simulink model "RM3ControlSim"  (R2015b)
settings: Solver=ode4  StartTime=0  StopTime=400  FixedStep=0.1  MaxStep=0.1  RelTol=1e-3
values from neighbouring files (symbols this model uses):
  simu = simulationClass()    [wecSimInputFile.m]
  waves = waveClass('irregular')    [wecSimInputFile.m]
undefined symbols (not defined in the file or in its folder): body, constraint, plant, pto, X, Y, Z
libraries: nesl_utility x72, vrlib x24, sm_lib x24, WECSim_Lib x3, simulink x2
(part 4 of 6)

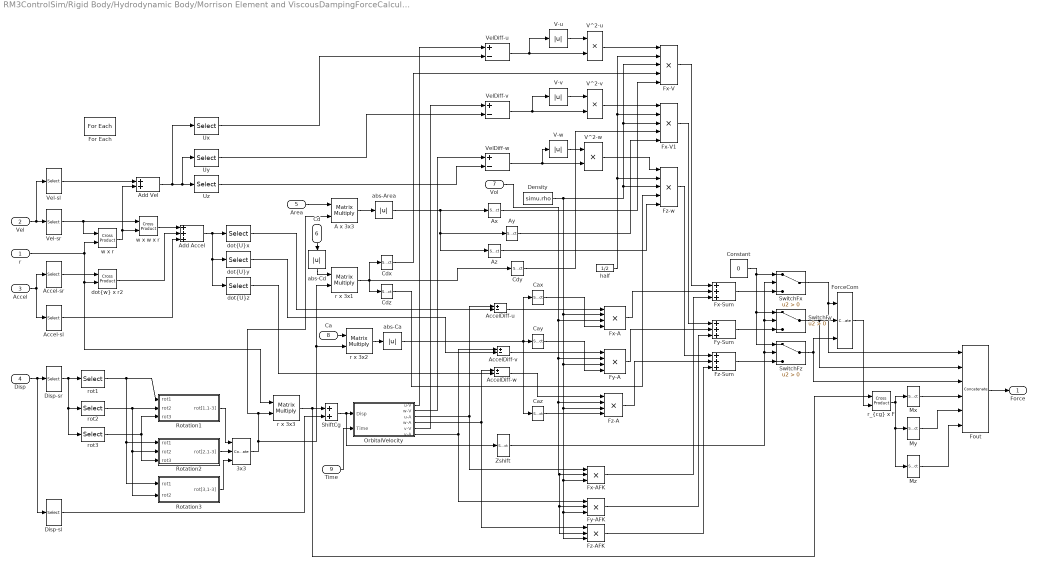
== system RM3ControlSim/Rigid Body/Hydrodynamic Body/Morrison Element and ViscousDampingForceCalculation/Morrison Element Variant Subsystem/Morrison Element On/Regular Wave Morison Force/MorrisonElements ==
  r : Inport  Partition=on  PartitionDimension=1  PartitionWidth=1
  Vel : Inport  Port=2
  Accel : Inport  Port=3
  Disp : Inport  Port=4
  Area : Inport  Port=5  Partition=on  PartitionDimension=1  PartitionWidth=1
  Cd : Inport  Port=6  Partition=on  PartitionDimension=1  PartitionWidth=1
  Vol : Inport  Port=7  Partition=on  PartitionDimension=1  PartitionWidth=1
  Ca : Inport  Port=8  Partition=on  PartitionDimension=1  PartitionWidth=1
  Time : Inport  Port=9
  3x3 : Concatenate  NumInputs=3  Mode=Multidimensional array
  A x 3x3 : Product  Multiplication=Matrix(*)
  Accel-sl : Selector  InputPortWidth=6  IndexOptions=Index vector (dialog)  Indices=[1 2 3]  OutputSizes=1
  Accel-sr : Selector  InputPortWidth=6  IndexOptions=Index vector (dialog)  Indices=[4 5 6]  OutputSizes=1
  AccelDiff-u : Sum  Inputs=+-
  AccelDiff-v : Sum  Inputs=+-
  AccelDiff-w : Sum  Inputs=+-
  Add Accel : Sum  Inputs=+++
  Add Vel : Sum
  Ax : Selector  InputPortWidth=3  IndexOptions=Index vector (dialog)  Indices=[1]  OutputSizes=1
  Ay : Selector  InputPortWidth=3  IndexOptions=Index vector (dialog)  Indices=[2]  OutputSizes=1
  Az : Selector  InputPortWidth=3  IndexOptions=Index vector (dialog)  Indices=[3]  OutputSizes=1
  Cax : Selector  InputPortWidth=3  IndexOptions=Index vector (dialog)  Indices=[1]  OutputSizes=1
  Cay : Selector  InputPortWidth=3  IndexOptions=Index vector (dialog)  Indices=[2]  OutputSizes=1
  Caz : Selector  InputPortWidth=3  IndexOptions=Index vector (dialog)  Indices=[3]  OutputSizes=1
  Cdx : Selector  InputPortWidth=3  IndexOptions=Index vector (dialog)  Indices=[1]  OutputSizes=1
  Cdy : Selector  InputPortWidth=3  IndexOptions=Index vector (dialog)  Indices=[2]  OutputSizes=1
  Cdz : Selector  InputPortWidth=3  IndexOptions=Index vector (dialog)  Indices=[3]  OutputSizes=1
  Constant : Constant  Value=0
  Density : Constant  Value=simu.rho
  Disp-sl : Selector  InputPortWidth=6  IndexOptions=Index vector (dialog)  Indices=[1 2 3]  OutputSizes=1
  Disp-sr : Selector  InputPortWidth=6  IndexOptions=Index vector (dialog)  Indices=[4 5 6]  OutputSizes=1
  For Each : ForEach  DisableCoverage=on  IndexMode=One-based
  ForceCom : Concatenate  NumInputs=3  ConcatenateDimension=2
  Fout : Concatenate  NumInputs=6  Mode=Multidimensional array  ConcatenateDimension=2
  Fx-A : Product  Inputs=4
  Fx-AFK : Product  Inputs=3
  Fx-Sum : Sum  Inputs=+++
  Fx-V : Product  Inputs=5
  Fx-V1 : Product  Inputs=5
  Fy-A : Product  Inputs=4
  Fy-AFK : Product  Inputs=3
  Fy-Sum : Sum  Inputs=+++
  Fz-A : Product  Inputs=4
  Fz-AFK : Product  Inputs=3
  Fz-Sum : Sum  Inputs=+++
  Fz-w : Product  Inputs=5
  Mx : Selector  InputPortWidth=3  IndexOptions=Index vector (dialog)  Indices=[1]  OutputSizes=1
  My : Selector  InputPortWidth=3  IndexOptions=Index vector (dialog)  Indices=[2]  OutputSizes=1
  Mz : Selector  InputPortWidth=3  IndexOptions=Index vector (dialog)  Indices=[3]  OutputSizes=1
  OrbitalVelocity : Subsystem
  Rotation1 : Subsystem
  Rotation2 : Subsystem
  Rotation3 : Subsystem
  ShiftCg : Sum
  SwitchFx : Switch  Criteria=u2 > Threshold
  SwitchFy : Switch  Criteria=u2 > Threshold
  SwitchFz : Switch  Criteria=u2 > Threshold
  Ux : Selector  InputPortWidth=3  IndexOptions=Index vector (dialog)  Indices=[1]  OutputSizes=1
  Uy : Selector  InputPortWidth=3  IndexOptions=Index vector (dialog)  Indices=[2]  OutputSizes=1
  Uz : Selector  InputPortWidth=3  IndexOptions=Index vector (dialog)  Indices=[3]  OutputSizes=1
  V-u : Abs
  V-v : Abs
  V-w : Abs
  V^2-u : Product
  V^2-v : Product
  V^2-w : Product
  Vel-sl : Selector  InputPortWidth=6  IndexOptions=Index vector (dialog)  Indices=[1 2 3]  OutputSizes=1
  "Vel-sr " : Selector  InputPortWidth=6  IndexOptions=Index vector (dialog)  Indices=[4 5 6]  OutputSizes=1
  VelDiff-u : Sum  Inputs=+-
  VelDiff-v : Sum  Inputs=+-
  VelDiff-w : Sum  Inputs=+-
  Zshift : Selector  InputPortWidth=3  IndexOptions=Index vector (dialog)  Indices=[3]  OutputSizes=1
  abs-Area : Abs
  abs-Ca : Abs
  abs-Cd : Abs
  "dot{U}x" : Selector  InputPortWidth=3  IndexOptions=Index vector (dialog)  Indices=[1]  OutputSizes=1
  "dot{U}y" : Selector  InputPortWidth=3  IndexOptions=Index vector (dialog)  Indices=[2]  OutputSizes=1
  "dot{U}z" : Selector  InputPortWidth=3  IndexOptions=Index vector (dialog)  Indices=[3]  OutputSizes=1
  "dot{w} x r2" : vrlib/Utilities/Cross Product
  half : Constant  Value=1/2
  r x 3x1 : Product  Multiplication=Matrix(*)
  r x 3x2 : Product  Multiplication=Matrix(*)
  r x 3x3 : Product  Multiplication=Matrix(*)
  "r_{cg} x F" : vrlib/Utilities/Cross Product
  rot1 : Selector  InputPortWidth=3  IndexOptions=Index vector (dialog)  Indices=[1]  OutputSizes=1
  rot2 : Selector  InputPortWidth=3  IndexOptions=Index vector (dialog)  Indices=[2]  OutputSizes=1
  rot3 : Selector  InputPortWidth=3  IndexOptions=Index vector (dialog)  Indices=[3]  OutputSizes=1
  w x r : vrlib/Utilities/Cross Product
  w x w x r : vrlib/Utilities/Cross Product
  Force : Outport  PortDimensions=[1 6]  ConcatenationDimension=1
  wires:
  Time/1 -> OrbitalVelocity/2(Time)
  abs-Cd/1 -> r x 3x1/1
  abs-Ca/1 -> Caz/1, Cay/1, Cax/1
  V-w/1 -> V^2-w/1
  Constant/1 -> SwitchFx/1, SwitchFz/1, SwitchFy/1
  Fx-V1/1 -> Fy-Sum/1
  Fy-A/1 -> Fy-Sum/2
  Cay/1 -> Fy-A/4
  AccelDiff-v/1 -> Fy-A/1
  Fy-AFK/1 -> Fy-Sum/3
  Fy-Sum/1 -> SwitchFy/3
  SwitchFy/1 -> ForceCom/2, Fout/2
  Cdy/1 -> Fx-V1/4
  Ay/1 -> Fx-V1/5
  OrbitalVelocity/5(v-V) -> VelDiff-v/1
  VelDiff-v/1 -> V^2-v/2, V-v/1
  V-v/1 -> V^2-v/1
  V^2-v/1 -> Fx-V1/1
  OrbitalVelocity/6(v-A) -> Fy-AFK/1, AccelDiff-v/1
  r x 3x2/1 -> abs-Ca/1
  Ca/1 -> r x 3x2/1
  r x 3x1/1 -> Cdx/1, Cdz/1, Cdy/1
  Cd/1 -> abs-Cd/1
  Cax/1 -> Fx-A/4
  Caz/1 -> Fz-A/4
  Fout/1 -> Force/1
  ForceCom/1 -> "r_{cg} x F"/2
  abs-Area/1 -> Ax/1, Az/1, Ay/1
  A x 3x3/1 -> abs-Area/1
  Cdz/1 -> Fz-w/4
  Cdx/1 -> Fx-V/4
  Ax/1 -> Fx-V/5
  Area/1 -> A x 3x3/1
  Az/1 -> Fz-w/5
  Fz-Sum/1 -> SwitchFz/3
  Fx-Sum/1 -> SwitchFx/3
  SwitchFx/1 -> ForceCom/1, Fout/1
  SwitchFz/1 -> Fout/3, ForceCom/3
  Zshift/1 -> SwitchFz/2, SwitchFx/2, SwitchFy/2
  VelDiff-u/1 -> V^2-u/2, V-u/1
  V-u/1 -> V^2-u/1
  3x3/1 -> r x 3x1/2, r x 3x2/2, r x 3x3/2, A x 3x3/2
  Mz/1 -> Fout/6
  My/1 -> Fout/5
  Mx/1 -> Fout/4
  "r_{cg} x F"/1 -> Mx/1, My/1, Mz/1
  Fz-AFK/1 -> Fz-Sum/3
  Fz-A/1 -> Fz-Sum/2
  Fz-w/1 -> Fz-Sum/1
  Fx-AFK/1 -> Fx-Sum/3
  Fx-A/1 -> Fx-Sum/2
  Fx-V/1 -> Fx-Sum/1
  OrbitalVelocity/4(w-A) -> AccelDiff-w/1, Fz-AFK/1
  AccelDiff-w/1 -> Fz-A/1
  Vol/1 -> Fx-A/3, Fz-A/2, Fx-AFK/2, Fz-AFK/2, Fy-AFK/2, Fy-A/2
  AccelDiff-u/1 -> Fx-A/1
  V^2-w/1 -> Fz-w/1
  Density/1 -> Fx-V/3, Fx-V1/3, Fz-w/3, Fx-A/2, Fz-A/3, Fx-AFK/3, Fz-AFK/3, Fy-AFK/3, Fy-A/3
  half/1 -> Fx-V/2, Fx-V1/2, Fz-w/2
  V^2-u/1 -> Fx-V/1
  VelDiff-w/1 -> V^2-w/2, V-w/1
  OrbitalVelocity/2(w-V) -> VelDiff-w/1
  OrbitalVelocity/1(u-V) -> VelDiff-u/1
  Uz/1 -> VelDiff-w/2
  Ux/1 -> VelDiff-u/2
  Uy/1 -> VelDiff-v/2
  Add Vel/1 -> Ux/1, Uz/1, Uy/1
  "dot{U}z"/1 -> AccelDiff-w/2
  OrbitalVelocity/3(u-A) -> Fx-AFK/1, AccelDiff-u/1
  "dot{U}x"/1 -> AccelDiff-u/2
  "dot{U}y"/1 -> AccelDiff-v/2
  ShiftCg/1 -> OrbitalVelocity/1(Disp), Zshift/1
  Disp-sl/1 -> ShiftCg/2
  r x 3x3/1 -> ShiftCg/1, "r_{cg} x F"/1
  Rotation3/1(rot[3,1-3]) -> 3x3/3
  Rotation1/1(rot[1,1-3]) -> 3x3/1
  Rotation2/1(rot[2,1-3]) -> 3x3/2
  rot2/1 -> Rotation1/2(rot2), Rotation2/2(rot2), Rotation3/2(rot2)
  rot1/1 -> Rotation1/1(rot1), Rotation2/1(rot1), Rotation3/1(rot1)
  rot3/1 -> Rotation1/3(rot3), Rotation2/3(rot3)
  Disp-sr/1 -> rot1/1, rot2/1, rot3/1
  Disp/1 -> Disp-sr/1, Disp-sl/1
  Vel-sl/1 -> Add Vel/1
  Add Accel/1 -> "dot{U}x"/1, "dot{U}y"/1, "dot{U}z"/1
  Accel-sl/1 -> Add Accel/3
  "dot{w} x r2"/1 -> Add Accel/2
  Accel-sr/1 -> "dot{w} x r2"/1
  Accel/1 -> Accel-sr/1, Accel-sl/1
  r/1 -> w x r/2, "dot{w} x r2"/2, r x 3x3/1
  "Vel-sr "/1 -> w x r/1, w x w x r/1
  w x w x r/1 -> Add Accel/1
  w x r/1 -> w x w x r/2, Add Vel/2
  Vel/1 -> "Vel-sr "/1, Vel-sl/1

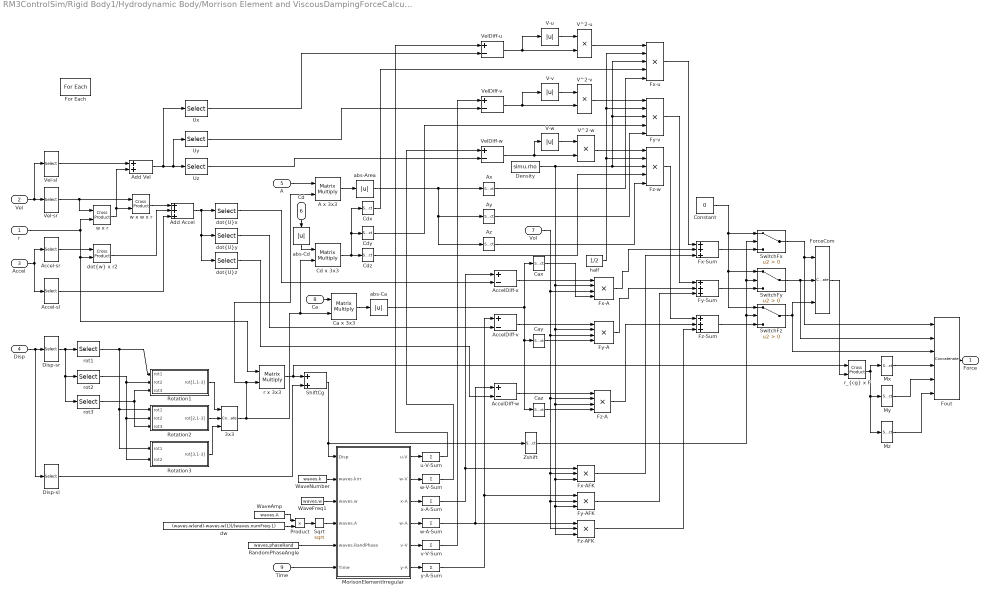
== system RM3ControlSim/Rigid Body1/Hydrodynamic Body/Morrison Element and ViscousDampingForceCalculation/Morrison Element Variant Subsystem/Morrison Element On/Irregular Wave Morison Force/MorrisonElements ==
  r : Inport  Partition=on  PartitionDimension=1  PartitionWidth=1
  Vel : Inport  Port=2
  Accel : Inport  Port=3
  Disp : Inport  Port=4
  A : Inport  Port=5  Partition=on  PartitionDimension=1  PartitionWidth=1
  Cd : Inport  Port=6  Partition=on  PartitionDimension=1  PartitionWidth=1
  Vol : Inport  Port=7  Partition=on  PartitionDimension=1  PartitionWidth=1
  Ca : Inport  Port=8  Partition=on  PartitionDimension=1  PartitionWidth=1
  Time : Inport  Port=9
  3x3 : Concatenate  NumInputs=3  Mode=Multidimensional array
  A x 3x3 : Product  Multiplication=Matrix(*)
  Accel-sl : Selector  InputPortWidth=6  IndexOptions=Index vector (dialog)  Indices=[1 2 3]  OutputSizes=1
  Accel-sr : Selector  InputPortWidth=6  IndexOptions=Index vector (dialog)  Indices=[4 5 6]  OutputSizes=1
  AccelDiff-v : Sum  Inputs=+-
  AccelDiff-w : Sum  Inputs=+-
  AccelDiff-x : Sum  Inputs=+-
  Add Accel : Sum  Inputs=+++
  Add Vel : Sum
  Ax : Selector  InputPortWidth=3  IndexOptions=Index vector (dialog)  Indices=[1]  OutputSizes=1
  Ay : Selector  InputPortWidth=3  IndexOptions=Index vector (dialog)  Indices=[2]  OutputSizes=1
  Az : Selector  InputPortWidth=3  IndexOptions=Index vector (dialog)  Indices=[3]  OutputSizes=1
  Ca x 3x3 : Product  Multiplication=Matrix(*)
  Cax : Selector  InputPortWidth=3  IndexOptions=Index vector (dialog)  Indices=[1]  OutputSizes=1
  Cay : Selector  InputPortWidth=3  IndexOptions=Index vector (dialog)  Indices=[2]  OutputSizes=1
  Caz : Selector  InputPortWidth=3  IndexOptions=Index vector (dialog)  Indices=[3]  OutputSizes=1
  Cd x 3x3 : Product  Multiplication=Matrix(*)
  Cdx : Selector  InputPortWidth=3  IndexOptions=Index vector (dialog)  Indices=[1]  OutputSizes=1
  Cdy : Selector  InputPortWidth=3  IndexOptions=Index vector (dialog)  Indices=[2]  OutputSizes=1
  Cdz : Selector  InputPortWidth=3  IndexOptions=Index vector (dialog)  Indices=[3]  OutputSizes=1
  Constant : Constant  Value=0
  Density : Constant  Value=simu.rho
  Disp-sl : Selector  InputPortWidth=6  IndexOptions=Index vector (dialog)  Indices=[1 2 3]  OutputSizes=1
  Disp-sr : Selector  InputPortWidth=6  IndexOptions=Index vector (dialog)  Indices=[4 5 6]  OutputSizes=1
  For Each : ForEach  DisableCoverage=on  IndexMode=One-based
  ForceCom : Concatenate  NumInputs=3  ConcatenateDimension=2
  Fout : Concatenate  NumInputs=6  Mode=Multidimensional array  ConcatenateDimension=2
  Fx-A : Product  Inputs=4
  Fx-AFK : Product  Inputs=3
  Fx-Sum : Sum  Inputs=+++
  Fx-u : Product  Inputs=5
  Fy-A : Product  Inputs=4
  Fy-AFK : Product  Inputs=3
  Fy-Sum : Sum  Inputs=+++
  Fy-v : Product  Inputs=5
  Fz-A : Product  Inputs=4
  Fz-AFK : Product  Inputs=3
  Fz-Sum : Sum  Inputs=+++
  Fz-w : Product  Inputs=5
  MorisonElementIrregular : Subsystem  TreatAsAtomicUnit=on
  Mx : Selector  InputPortWidth=3  IndexOptions=Index vector (dialog)  Indices=[1]  OutputSizes=1
  My : Selector  InputPortWidth=3  IndexOptions=Index vector (dialog)  Indices=[2]  OutputSizes=1
  Mz : Selector  InputPortWidth=3  IndexOptions=Index vector (dialog)  Indices=[3]  OutputSizes=1
  Product : Product
  RandomPhaseAngle : Constant  Value=waves.phaseRand  VectorParams1D=off
  Rotation1 : Subsystem
  Rotation2 : Subsystem
  Rotation3 : Subsystem
  ShiftCg : Sum
  Sqrt : Sqrt  SaturateOnIntegerOverflow=on
  SwitchFx : Switch  Criteria=u2 > Threshold
  SwitchFy : Switch  Criteria=u2 > Threshold
  SwitchFz : Switch  Criteria=u2 > Threshold
  Ux : Selector  InputPortWidth=3  IndexOptions=Index vector (dialog)  Indices=[1]  OutputSizes=1
  Uy : Selector  InputPortWidth=3  IndexOptions=Index vector (dialog)  Indices=[2]  OutputSizes=1
  Uz : Selector  InputPortWidth=3  IndexOptions=Index vector (dialog)  Indices=[3]  OutputSizes=1
  V-u : Abs
  V-v : Abs
  V-w : Abs
  V^2-u : Product
  V^2-v : Product
  V^2-w : Product
  Vel-sl : Selector  InputPortWidth=6  IndexOptions=Index vector (dialog)  Indices=[1 2 3]  OutputSizes=1
  "Vel-sr " : Selector  InputPortWidth=6  IndexOptions=Index vector (dialog)  Indices=[4 5 6]  OutputSizes=1
  VelDiff-u : Sum  Inputs=+-
  VelDiff-v : Sum  Inputs=+-
  VelDiff-w : Sum  Inputs=+-
  WaveAmp : Constant  Value=waves.A  VectorParams1D=off
  WaveFreq1 : Constant  Value=waves.w  VectorParams1D=off
  WaveNumber : Constant  Value=waves.k  VectorParams1D=off
  Zshift : Selector  InputPortWidth=3  IndexOptions=Index vector (dialog)  Indices=[3]  OutputSizes=1
  abs-Area : Abs
  abs-Ca : Abs
  abs-Cd : Abs
  "dot{U}x" : Selector  InputPortWidth=3  IndexOptions=Index vector (dialog)  Indices=[1]  OutputSizes=1
  "dot{U}y" : Selector  InputPortWidth=3  IndexOptions=Index vector (dialog)  Indices=[2]  OutputSizes=1
  "dot{U}z" : Selector  InputPortWidth=3  IndexOptions=Index vector (dialog)  Indices=[3]  OutputSizes=1
  "dot{w} x r2" : vrlib/Utilities/Cross Product
  dw : Constant  Value=(waves.w(end)-waves.w(1))/(waves.numFreq-1)  VectorParams1D=off
  half : Constant  Value=1/2
  r x 3x3 : Product  Multiplication=Matrix(*)
  "r_{cg} x F" : vrlib/Utilities/Cross Product
  rot1 : Selector  InputPortWidth=3  IndexOptions=Index vector (dialog)  Indices=[1]  OutputSizes=1
  rot2 : Selector  InputPortWidth=3  IndexOptions=Index vector (dialog)  Indices=[2]  OutputSizes=1
  rot3 : Selector  InputPortWidth=3  IndexOptions=Index vector (dialog)  Indices=[3]  OutputSizes=1
  u-V-Sum : Sum  Inputs=+  CollapseMode=Specified dimension
  v-V-Sum : Sum  Inputs=+  CollapseMode=Specified dimension
  w x r : vrlib/Utilities/Cross Product
  w x w x r : vrlib/Utilities/Cross Product
  w-A-Sum : Sum  Inputs=+  CollapseMode=Specified dimension
  w-V-Sum : Sum  Inputs=+  CollapseMode=Specified dimension
  x-A-Sum : Sum  Inputs=+  CollapseMode=Specified dimension
  y-A-Sum : Sum  Inputs=+  CollapseMode=Specified dimension
  Force : Outport  PortDimensions=[1 6]  ConcatenationDimension=1
  wires:
  Time/1 -> MorisonElementIrregular/6(Time)
  abs-Cd/1 -> Cd x 3x3/1
  abs-Ca/1 -> Cay/1, Caz/1, Cax/1
  Fy-AFK/1 -> Fy-Sum/3
  Fy-A/1 -> Fy-Sum/2
  AccelDiff-v/1 -> Fy-A/1
  Cay/1 -> Fy-A/4
  y-A-Sum/1 -> AccelDiff-v/1, Fy-AFK/1
  Fy-v/1 -> Fy-Sum/1
  Fy-Sum/1 -> SwitchFy/3
  SwitchFy/1 -> ForceCom/2, Fout/2
  Cdy/1 -> Fy-v/4
  Ay/1 -> Fy-v/5
  V^2-v/1 -> Fy-v/1
  v-V-Sum/1 -> VelDiff-v/1
  V-v/1 -> V^2-v/1
  VelDiff-v/1 -> V^2-v/2, V-v/1
  V-w/1 -> V^2-w/1
  MorisonElementIrregular/6(y-A) -> y-A-Sum/1
  MorisonElementIrregular/5(v-V) -> v-V-Sum/1
  V-u/1 -> V^2-u/1
  MorisonElementIrregular/4(w-A) -> w-A-Sum/1
  MorisonElementIrregular/3(x-A) -> x-A-Sum/1
  MorisonElementIrregular/2(w-V) -> w-V-Sum/1
  Sqrt/1 -> MorisonElementIrregular/4(waves.A)
  Product/1 -> Sqrt/1
  dw/1 -> Product/2
  WaveAmp/1 -> Product/1
  MorisonElementIrregular/1(u-V) -> u-V-Sum/1
  RandomPhaseAngle/1 -> MorisonElementIrregular/5(waves.RandPhase)
  WaveFreq1/1 -> MorisonElementIrregular/3(waves.w)
  WaveNumber/1 -> MorisonElementIrregular/2(waves.kirr)
  Ca x 3x3/1 -> abs-Ca/1
  Ca/1 -> Ca x 3x3/1
  Cd x 3x3/1 -> Cdx/1, Cdy/1, Cdz/1
  Cd/1 -> abs-Cd/1
  Cax/1 -> Fx-A/4
  Caz/1 -> Fz-A/4
  Fout/1 -> Force/1
  ForceCom/1 -> "r_{cg} x F"/2
  abs-Area/1 -> Ax/1, Az/1, Ay/1
  A x 3x3/1 -> abs-Area/1
  Cdz/1 -> Fz-w/4
  Cdx/1 -> Fx-u/4
  Ax/1 -> Fx-u/5
  A/1 -> A x 3x3/1
  Az/1 -> Fz-w/5
  Fz-Sum/1 -> SwitchFz/3
  Fx-Sum/1 -> SwitchFx/3
  SwitchFx/1 -> ForceCom/1, Fout/1
  SwitchFz/1 -> Fout/3, ForceCom/3
  Zshift/1 -> SwitchFz/2, SwitchFx/2, SwitchFy/2
  VelDiff-u/1 -> V^2-u/2, V-u/1
  3x3/1 -> Cd x 3x3/2, Ca x 3x3/2, r x 3x3/2, A x 3x3/2
  Mz/1 -> Fout/6
  My/1 -> Fout/5
  Mx/1 -> Fout/4
  "r_{cg} x F"/1 -> Mx/1, My/1, Mz/1
  Constant/1 -> SwitchFx/1, SwitchFz/1, SwitchFy/1
  Fz-AFK/1 -> Fz-Sum/3
  Fz-A/1 -> Fz-Sum/2
  Fz-w/1 -> Fz-Sum/1
  Fx-AFK/1 -> Fx-Sum/3
  Fx-A/1 -> Fx-Sum/2
  Fx-u/1 -> Fx-Sum/1
  w-A-Sum/1 -> Fz-AFK/1, AccelDiff-w/1
  AccelDiff-w/1 -> Fz-A/1
  Vol/1 -> Fx-A/3, Fz-A/2, Fx-AFK/2, Fz-AFK/2, Fy-AFK/2, Fy-A/3
  AccelDiff-x/1 -> Fx-A/1
  V^2-w/1 -> Fz-w/1
  Density/1 -> Fz-w/3, Fx-u/3, Fy-v/3, Fx-A/2, Fz-A/3, Fx-AFK/3, Fz-AFK/3, Fy-AFK/3, Fy-A/2
  half/1 -> Fx-u/2, Fy-v/2, Fz-w/2
  V^2-u/1 -> Fx-u/1
  VelDiff-w/1 -> V-w/1, V^2-w/2
  w-V-Sum/1 -> VelDiff-w/1
  u-V-Sum/1 -> VelDiff-u/1
  Uz/1 -> VelDiff-w/2
  Ux/1 -> VelDiff-u/2
  Uy/1 -> VelDiff-v/2
  Add Vel/1 -> Uz/1, Uy/1, Ux/1
  "dot{U}z"/1 -> AccelDiff-w/2
  x-A-Sum/1 -> AccelDiff-x/1, Fx-AFK/1
  "dot{U}x"/1 -> AccelDiff-x/2
  "dot{U}y"/1 -> AccelDiff-v/2
  ShiftCg/1 -> Zshift/1, MorisonElementIrregular/1(Disp)
  Disp-sl/1 -> ShiftCg/2
  r x 3x3/1 -> ShiftCg/1, "r_{cg} x F"/1
  Rotation3/1(rot[3,1-3]) -> 3x3/3
  Rotation1/1(rot[1,1-3]) -> 3x3/1
  Rotation2/1(rot[2,1-3]) -> 3x3/2
  rot2/1 -> Rotation1/2(rot2), Rotation2/2(rot2), Rotation3/2(rot2)
  rot1/1 -> Rotation1/1(rot1), Rotation2/1(rot1), Rotation3/1(rot1)
  rot3/1 -> Rotation1/3(rot3), Rotation2/3(rot3)
  Disp-sr/1 -> rot1/1, rot2/1, rot3/1
  Disp/1 -> Disp-sr/1, Disp-sl/1
  Vel-sl/1 -> Add Vel/1
  Add Accel/1 -> "dot{U}x"/1, "dot{U}y"/1, "dot{U}z"/1
  Accel-sl/1 -> Add Accel/3
  "dot{w} x r2"/1 -> Add Accel/2
  Accel-sr/1 -> "dot{w} x r2"/1
  Accel/1 -> Accel-sr/1, Accel-sl/1
  r/1 -> w x r/2, "dot{w} x r2"/2, r x 3x3/1
  "Vel-sr "/1 -> w x r/1, w x w x r/1
  w x w x r/1 -> Add Accel/1
  w x r/1 -> w x w x r/2, Add Vel/2
  Vel/1 -> "Vel-sr "/1, Vel-sl/1

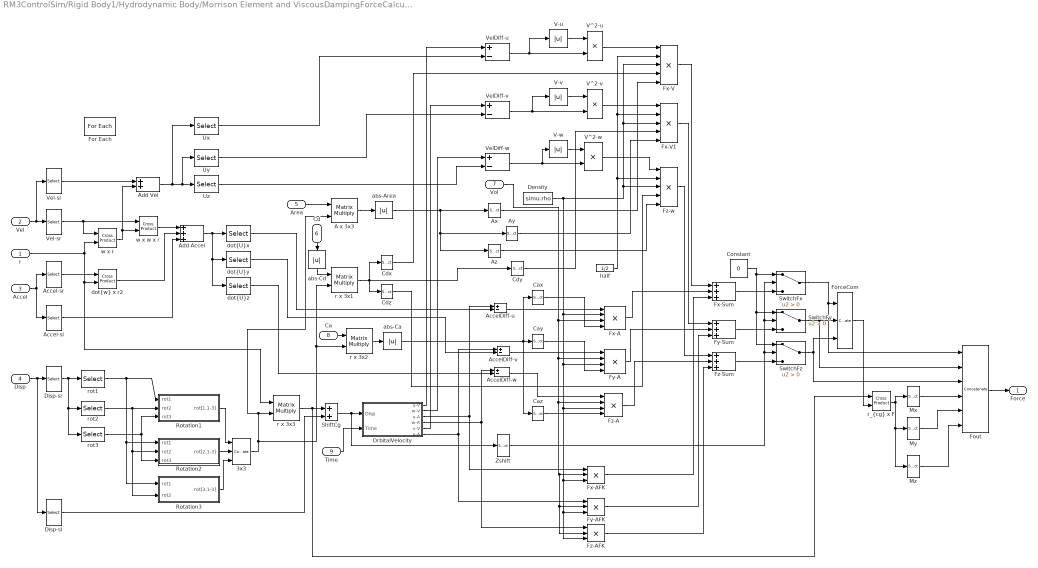
== system RM3ControlSim/Rigid Body1/Hydrodynamic Body/Morrison Element and ViscousDampingForceCalculation/Morrison Element Variant Subsystem/Morrison Element On/No Wave Morison Force/MorrisonElements ==
  r : Inport  Partition=on  PartitionDimension=1  PartitionWidth=1
  Vel : Inport  Port=2
  Accel : Inport  Port=3
  Disp : Inport  Port=4
  Area : Inport  Port=5  Partition=on  PartitionDimension=1  PartitionWidth=1
  Cd : Inport  Port=6  Partition=on  PartitionDimension=1  PartitionWidth=1
  Vol : Inport  Port=7  Partition=on  PartitionDimension=1  PartitionWidth=1
  Ca : Inport  Port=8  Partition=on  PartitionDimension=1  PartitionWidth=1
  Time : Inport  Port=9
  3x3 : Concatenate  NumInputs=3  Mode=Multidimensional array
  A x 3x3 : Product  Multiplication=Matrix(*)
  Accel-sl : Selector  InputPortWidth=6  IndexOptions=Index vector (dialog)  Indices=[1 2 3]  OutputSizes=1
  Accel-sr : Selector  InputPortWidth=6  IndexOptions=Index vector (dialog)  Indices=[4 5 6]  OutputSizes=1
  AccelDiff-u : Sum  Inputs=+-
  AccelDiff-v : Sum  Inputs=+-
  AccelDiff-w : Sum  Inputs=+-
  Add Accel : Sum  Inputs=+++
  Add Vel : Sum
  Ax : Selector  InputPortWidth=3  IndexOptions=Index vector (dialog)  Indices=[1]  OutputSizes=1
  Ay : Selector  InputPortWidth=3  IndexOptions=Index vector (dialog)  Indices=[2]  OutputSizes=1
  Az : Selector  InputPortWidth=3  IndexOptions=Index vector (dialog)  Indices=[3]  OutputSizes=1
  Cax : Selector  InputPortWidth=3  IndexOptions=Index vector (dialog)  Indices=[1]  OutputSizes=1
  Cay : Selector  InputPortWidth=3  IndexOptions=Index vector (dialog)  Indices=[2]  OutputSizes=1
  Caz : Selector  InputPortWidth=3  IndexOptions=Index vector (dialog)  Indices=[3]  OutputSizes=1
  Cdx : Selector  InputPortWidth=3  IndexOptions=Index vector (dialog)  Indices=[1]  OutputSizes=1
  Cdy : Selector  InputPortWidth=3  IndexOptions=Index vector (dialog)  Indices=[2]  OutputSizes=1
  Cdz : Selector  InputPortWidth=3  IndexOptions=Index vector (dialog)  Indices=[3]  OutputSizes=1
  Constant : Constant  Value=0
  Density : Constant  Value=simu.rho
  Disp-sl : Selector  InputPortWidth=6  IndexOptions=Index vector (dialog)  Indices=[1 2 3]  OutputSizes=1
  Disp-sr : Selector  InputPortWidth=6  IndexOptions=Index vector (dialog)  Indices=[4 5 6]  OutputSizes=1
  For Each : ForEach  DisableCoverage=on  IndexMode=One-based
  ForceCom : Concatenate  NumInputs=3  ConcatenateDimension=2
  Fout : Concatenate  NumInputs=6  Mode=Multidimensional array  ConcatenateDimension=2
  Fx-A : Product  Inputs=4
  Fx-AFK : Product  Inputs=3
  Fx-Sum : Sum  Inputs=+++
  Fx-V : Product  Inputs=5
  Fx-V1 : Product  Inputs=5
  Fy-A : Product  Inputs=4
  Fy-AFK : Product  Inputs=3
  Fy-Sum : Sum  Inputs=+++
  Fz-A : Product  Inputs=4
  Fz-AFK : Product  Inputs=3
  Fz-Sum : Sum  Inputs=+++
  Fz-w : Product  Inputs=5
  Mx : Selector  InputPortWidth=3  IndexOptions=Index vector (dialog)  Indices=[1]  OutputSizes=1
  My : Selector  InputPortWidth=3  IndexOptions=Index vector (dialog)  Indices=[2]  OutputSizes=1
  Mz : Selector  InputPortWidth=3  IndexOptions=Index vector (dialog)  Indices=[3]  OutputSizes=1
  OrbitalVelocity : Subsystem
  Rotation1 : Subsystem
  Rotation2 : Subsystem
  Rotation3 : Subsystem
  ShiftCg : Sum
  SwitchFx : Switch  Criteria=u2 > Threshold
  SwitchFy : Switch  Criteria=u2 > Threshold
  SwitchFz : Switch  Criteria=u2 > Threshold
  Ux : Selector  InputPortWidth=3  IndexOptions=Index vector (dialog)  Indices=[1]  OutputSizes=1
  Uy : Selector  InputPortWidth=3  IndexOptions=Index vector (dialog)  Indices=[2]  OutputSizes=1
  Uz : Selector  InputPortWidth=3  IndexOptions=Index vector (dialog)  Indices=[3]  OutputSizes=1
  V-u : Abs
  V-v : Abs
  V-w : Abs
  V^2-u : Product
  V^2-v : Product
  V^2-w : Product
  Vel-sl : Selector  InputPortWidth=6  IndexOptions=Index vector (dialog)  Indices=[1 2 3]  OutputSizes=1
  "Vel-sr " : Selector  InputPortWidth=6  IndexOptions=Index vector (dialog)  Indices=[4 5 6]  OutputSizes=1
  VelDiff-u : Sum  Inputs=+-
  VelDiff-v : Sum  Inputs=+-
  VelDiff-w : Sum  Inputs=+-
  Zshift : Selector  InputPortWidth=3  IndexOptions=Index vector (dialog)  Indices=[3]  OutputSizes=1
  abs-Area : Abs
  abs-Ca : Abs
  abs-Cd : Abs
  "dot{U}x" : Selector  InputPortWidth=3  IndexOptions=Index vector (dialog)  Indices=[1]  OutputSizes=1
  "dot{U}y" : Selector  InputPortWidth=3  IndexOptions=Index vector (dialog)  Indices=[2]  OutputSizes=1
  "dot{U}z" : Selector  InputPortWidth=3  IndexOptions=Index vector (dialog)  Indices=[3]  OutputSizes=1
  "dot{w} x r2" : vrlib/Utilities/Cross Product
  half : Constant  Value=1/2
  r x 3x1 : Product  Multiplication=Matrix(*)
  r x 3x2 : Product  Multiplication=Matrix(*)
  r x 3x3 : Product  Multiplication=Matrix(*)
  "r_{cg} x F" : vrlib/Utilities/Cross Product
  rot1 : Selector  InputPortWidth=3  IndexOptions=Index vector (dialog)  Indices=[1]  OutputSizes=1
  rot2 : Selector  InputPortWidth=3  IndexOptions=Index vector (dialog)  Indices=[2]  OutputSizes=1
  rot3 : Selector  InputPortWidth=3  IndexOptions=Index vector (dialog)  Indices=[3]  OutputSizes=1
  w x r : vrlib/Utilities/Cross Product
  w x w x r : vrlib/Utilities/Cross Product
  Force : Outport  PortDimensions=[1 6]  ConcatenationDimension=1
  wires:
  Time/1 -> OrbitalVelocity/2(Time)
  abs-Cd/1 -> r x 3x1/1
  abs-Ca/1 -> Caz/1, Cay/1, Cax/1
  V-w/1 -> V^2-w/1
  Constant/1 -> SwitchFx/1, SwitchFz/1, SwitchFy/1
  Fx-V1/1 -> Fy-Sum/1
  Fy-A/1 -> Fy-Sum/2
  Cay/1 -> Fy-A/4
  AccelDiff-v/1 -> Fy-A/1
  Fy-AFK/1 -> Fy-Sum/3
  Fy-Sum/1 -> SwitchFy/3
  SwitchFy/1 -> ForceCom/2, Fout/2
  Cdy/1 -> Fx-V1/4
  Ay/1 -> Fx-V1/5
  OrbitalVelocity/5(v-V) -> VelDiff-v/1
  VelDiff-v/1 -> V^2-v/2, V-v/1
  V-v/1 -> V^2-v/1
  V^2-v/1 -> Fx-V1/1
  OrbitalVelocity/6(v-A) -> Fy-AFK/1, AccelDiff-v/1
  r x 3x2/1 -> abs-Ca/1
  Ca/1 -> r x 3x2/1
  r x 3x1/1 -> Cdx/1, Cdz/1, Cdy/1
  Cd/1 -> abs-Cd/1
  Cax/1 -> Fx-A/4
  Caz/1 -> Fz-A/4
  Fout/1 -> Force/1
  ForceCom/1 -> "r_{cg} x F"/2
  abs-Area/1 -> Ax/1, Az/1, Ay/1
  A x 3x3/1 -> abs-Area/1
  Cdz/1 -> Fz-w/4
  Cdx/1 -> Fx-V/4
  Ax/1 -> Fx-V/5
  Area/1 -> A x 3x3/1
  Az/1 -> Fz-w/5
  Fz-Sum/1 -> SwitchFz/3
  Fx-Sum/1 -> SwitchFx/3
  SwitchFx/1 -> ForceCom/1, Fout/1
  SwitchFz/1 -> Fout/3, ForceCom/3
  Zshift/1 -> SwitchFz/2, SwitchFx/2, SwitchFy/2
  VelDiff-u/1 -> V^2-u/2, V-u/1
  V-u/1 -> V^2-u/1
  3x3/1 -> r x 3x1/2, r x 3x2/2, r x 3x3/2, A x 3x3/2
  Mz/1 -> Fout/6
  My/1 -> Fout/5
  Mx/1 -> Fout/4
  "r_{cg} x F"/1 -> Mx/1, My/1, Mz/1
  Fz-AFK/1 -> Fz-Sum/3
  Fz-A/1 -> Fz-Sum/2
  Fz-w/1 -> Fz-Sum/1
  Fx-AFK/1 -> Fx-Sum/3
  Fx-A/1 -> Fx-Sum/2
  Fx-V/1 -> Fx-Sum/1
  OrbitalVelocity/4(w-A) -> AccelDiff-w/1, Fz-AFK/1
  AccelDiff-w/1 -> Fz-A/1
  Vol/1 -> Fx-A/3, Fz-A/2, Fx-AFK/2, Fz-AFK/2, Fy-AFK/2, Fy-A/2
  AccelDiff-u/1 -> Fx-A/1
  V^2-w/1 -> Fz-w/1
  Density/1 -> Fx-V/3, Fx-V1/3, Fz-w/3, Fx-A/2, Fz-A/3, Fx-AFK/3, Fz-AFK/3, Fy-AFK/3, Fy-A/3
  half/1 -> Fx-V/2, Fx-V1/2, Fz-w/2
  V^2-u/1 -> Fx-V/1
  VelDiff-w/1 -> V^2-w/2, V-w/1
  OrbitalVelocity/2(w-V) -> VelDiff-w/1
  OrbitalVelocity/1(u-V) -> VelDiff-u/1
  Uz/1 -> VelDiff-w/2
  Ux/1 -> VelDiff-u/2
  Uy/1 -> VelDiff-v/2
  Add Vel/1 -> Ux/1, Uz/1, Uy/1
  "dot{U}z"/1 -> AccelDiff-w/2
  OrbitalVelocity/3(u-A) -> Fx-AFK/1, AccelDiff-u/1
  "dot{U}x"/1 -> AccelDiff-u/2
  "dot{U}y"/1 -> AccelDiff-v/2
  ShiftCg/1 -> OrbitalVelocity/1(Disp), Zshift/1
  Disp-sl/1 -> ShiftCg/2
  r x 3x3/1 -> ShiftCg/1, "r_{cg} x F"/1
  Rotation3/1(rot[3,1-3]) -> 3x3/3
  Rotation1/1(rot[1,1-3]) -> 3x3/1
  Rotation2/1(rot[2,1-3]) -> 3x3/2
  rot2/1 -> Rotation1/2(rot2), Rotation2/2(rot2), Rotation3/2(rot2)
  rot1/1 -> Rotation1/1(rot1), Rotation2/1(rot1), Rotation3/1(rot1)
  rot3/1 -> Rotation1/3(rot3), Rotation2/3(rot3)
  Disp-sr/1 -> rot1/1, rot2/1, rot3/1
  Disp/1 -> Disp-sr/1, Disp-sl/1
  Vel-sl/1 -> Add Vel/1
  Add Accel/1 -> "dot{U}x"/1, "dot{U}y"/1, "dot{U}z"/1
  Accel-sl/1 -> Add Accel/3
  "dot{w} x r2"/1 -> Add Accel/2
  Accel-sr/1 -> "dot{w} x r2"/1
  Accel/1 -> Accel-sr/1, Accel-sl/1
  r/1 -> w x r/2, "dot{w} x r2"/2, r x 3x3/1
  "Vel-sr "/1 -> w x r/1, w x w x r/1
  w x w x r/1 -> Add Accel/1
  w x r/1 -> w x w x r/2, Add Vel/2
  Vel/1 -> "Vel-sr "/1, Vel-sl/1

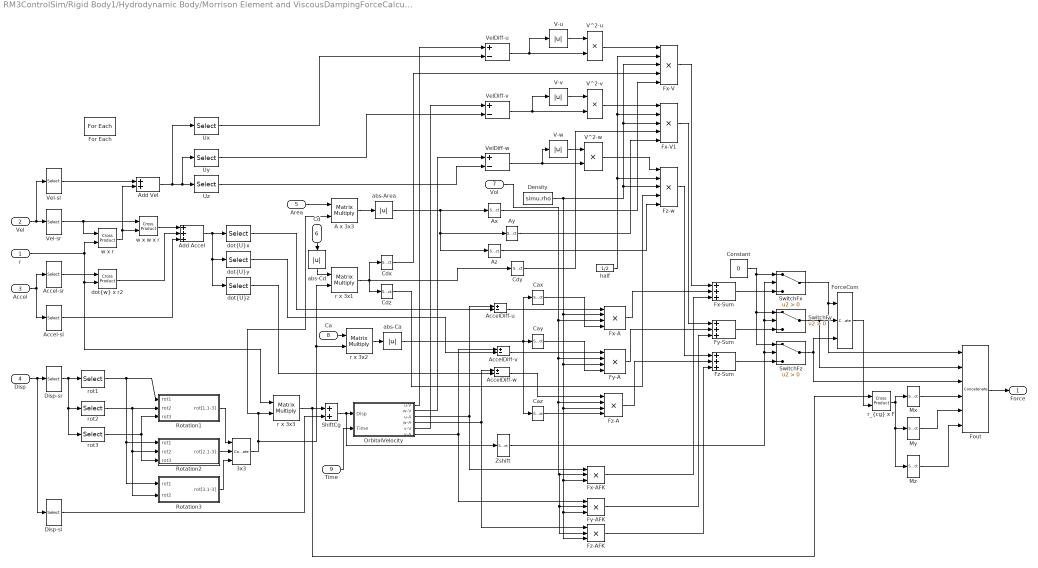
== system RM3ControlSim/Rigid Body1/Hydrodynamic Body/Morrison Element and ViscousDampingForceCalculation/Morrison Element Variant Subsystem/Morrison Element On/Regular Wave Morison Force/MorrisonElements ==
  r : Inport  Partition=on  PartitionDimension=1  PartitionWidth=1
  Vel : Inport  Port=2
  Accel : Inport  Port=3
  Disp : Inport  Port=4
  Area : Inport  Port=5  Partition=on  PartitionDimension=1  PartitionWidth=1
  Cd : Inport  Port=6  Partition=on  PartitionDimension=1  PartitionWidth=1
  Vol : Inport  Port=7  Partition=on  PartitionDimension=1  PartitionWidth=1
  Ca : Inport  Port=8  Partition=on  PartitionDimension=1  PartitionWidth=1
  Time : Inport  Port=9
  3x3 : Concatenate  NumInputs=3  Mode=Multidimensional array
  A x 3x3 : Product  Multiplication=Matrix(*)
  Accel-sl : Selector  InputPortWidth=6  IndexOptions=Index vector (dialog)  Indices=[1 2 3]  OutputSizes=1
  Accel-sr : Selector  InputPortWidth=6  IndexOptions=Index vector (dialog)  Indices=[4 5 6]  OutputSizes=1
  AccelDiff-u : Sum  Inputs=+-
  AccelDiff-v : Sum  Inputs=+-
  AccelDiff-w : Sum  Inputs=+-
  Add Accel : Sum  Inputs=+++
  Add Vel : Sum
  Ax : Selector  InputPortWidth=3  IndexOptions=Index vector (dialog)  Indices=[1]  OutputSizes=1
  Ay : Selector  InputPortWidth=3  IndexOptions=Index vector (dialog)  Indices=[2]  OutputSizes=1
  Az : Selector  InputPortWidth=3  IndexOptions=Index vector (dialog)  Indices=[3]  OutputSizes=1
  Cax : Selector  InputPortWidth=3  IndexOptions=Index vector (dialog)  Indices=[1]  OutputSizes=1
  Cay : Selector  InputPortWidth=3  IndexOptions=Index vector (dialog)  Indices=[2]  OutputSizes=1
  Caz : Selector  InputPortWidth=3  IndexOptions=Index vector (dialog)  Indices=[3]  OutputSizes=1
  Cdx : Selector  InputPortWidth=3  IndexOptions=Index vector (dialog)  Indices=[1]  OutputSizes=1
  Cdy : Selector  InputPortWidth=3  IndexOptions=Index vector (dialog)  Indices=[2]  OutputSizes=1
  Cdz : Selector  InputPortWidth=3  IndexOptions=Index vector (dialog)  Indices=[3]  OutputSizes=1
  Constant : Constant  Value=0
  Density : Constant  Value=simu.rho
  Disp-sl : Selector  InputPortWidth=6  IndexOptions=Index vector (dialog)  Indices=[1 2 3]  OutputSizes=1
  Disp-sr : Selector  InputPortWidth=6  IndexOptions=Index vector (dialog)  Indices=[4 5 6]  OutputSizes=1
  For Each : ForEach  DisableCoverage=on  IndexMode=One-based
  ForceCom : Concatenate  NumInputs=3  ConcatenateDimension=2
  Fout : Concatenate  NumInputs=6  Mode=Multidimensional array  ConcatenateDimension=2
  Fx-A : Product  Inputs=4
  Fx-AFK : Product  Inputs=3
  Fx-Sum : Sum  Inputs=+++
  Fx-V : Product  Inputs=5
  Fx-V1 : Product  Inputs=5
  Fy-A : Product  Inputs=4
  Fy-AFK : Product  Inputs=3
  Fy-Sum : Sum  Inputs=+++
  Fz-A : Product  Inputs=4
  Fz-AFK : Product  Inputs=3
  Fz-Sum : Sum  Inputs=+++
  Fz-w : Product  Inputs=5
  Mx : Selector  InputPortWidth=3  IndexOptions=Index vector (dialog)  Indices=[1]  OutputSizes=1
  My : Selector  InputPortWidth=3  IndexOptions=Index vector (dialog)  Indices=[2]  OutputSizes=1
  Mz : Selector  InputPortWidth=3  IndexOptions=Index vector (dialog)  Indices=[3]  OutputSizes=1
  OrbitalVelocity : Subsystem
  Rotation1 : Subsystem
  Rotation2 : Subsystem
  Rotation3 : Subsystem
  ShiftCg : Sum
  SwitchFx : Switch  Criteria=u2 > Threshold
  SwitchFy : Switch  Criteria=u2 > Threshold
  SwitchFz : Switch  Criteria=u2 > Threshold
  Ux : Selector  InputPortWidth=3  IndexOptions=Index vector (dialog)  Indices=[1]  OutputSizes=1
  Uy : Selector  InputPortWidth=3  IndexOptions=Index vector (dialog)  Indices=[2]  OutputSizes=1
  Uz : Selector  InputPortWidth=3  IndexOptions=Index vector (dialog)  Indices=[3]  OutputSizes=1
  V-u : Abs
  V-v : Abs
  V-w : Abs
  V^2-u : Product
  V^2-v : Product
  V^2-w : Product
  Vel-sl : Selector  InputPortWidth=6  IndexOptions=Index vector (dialog)  Indices=[1 2 3]  OutputSizes=1
  "Vel-sr " : Selector  InputPortWidth=6  IndexOptions=Index vector (dialog)  Indices=[4 5 6]  OutputSizes=1
  VelDiff-u : Sum  Inputs=+-
  VelDiff-v : Sum  Inputs=+-
  VelDiff-w : Sum  Inputs=+-
  Zshift : Selector  InputPortWidth=3  IndexOptions=Index vector (dialog)  Indices=[3]  OutputSizes=1
  abs-Area : Abs
  abs-Ca : Abs
  abs-Cd : Abs
  "dot{U}x" : Selector  InputPortWidth=3  IndexOptions=Index vector (dialog)  Indices=[1]  OutputSizes=1
  "dot{U}y" : Selector  InputPortWidth=3  IndexOptions=Index vector (dialog)  Indices=[2]  OutputSizes=1
  "dot{U}z" : Selector  InputPortWidth=3  IndexOptions=Index vector (dialog)  Indices=[3]  OutputSizes=1
  "dot{w} x r2" : vrlib/Utilities/Cross Product
  half : Constant  Value=1/2
  r x 3x1 : Product  Multiplication=Matrix(*)
  r x 3x2 : Product  Multiplication=Matrix(*)
  r x 3x3 : Product  Multiplication=Matrix(*)
  "r_{cg} x F" : vrlib/Utilities/Cross Product
  rot1 : Selector  InputPortWidth=3  IndexOptions=Index vector (dialog)  Indices=[1]  OutputSizes=1
  rot2 : Selector  InputPortWidth=3  IndexOptions=Index vector (dialog)  Indices=[2]  OutputSizes=1
  rot3 : Selector  InputPortWidth=3  IndexOptions=Index vector (dialog)  Indices=[3]  OutputSizes=1
  w x r : vrlib/Utilities/Cross Product
  w x w x r : vrlib/Utilities/Cross Product
  Force : Outport  PortDimensions=[1 6]  ConcatenationDimension=1
  wires:
  Time/1 -> OrbitalVelocity/2(Time)
  abs-Cd/1 -> r x 3x1/1
  abs-Ca/1 -> Caz/1, Cay/1, Cax/1
  V-w/1 -> V^2-w/1
  Constant/1 -> SwitchFx/1, SwitchFz/1, SwitchFy/1
  Fx-V1/1 -> Fy-Sum/1
  Fy-A/1 -> Fy-Sum/2
  Cay/1 -> Fy-A/4
  AccelDiff-v/1 -> Fy-A/1
  Fy-AFK/1 -> Fy-Sum/3
  Fy-Sum/1 -> SwitchFy/3
  SwitchFy/1 -> ForceCom/2, Fout/2
  Cdy/1 -> Fx-V1/4
  Ay/1 -> Fx-V1/5
  OrbitalVelocity/5(v-V) -> VelDiff-v/1
  VelDiff-v/1 -> V^2-v/2, V-v/1
  V-v/1 -> V^2-v/1
  V^2-v/1 -> Fx-V1/1
  OrbitalVelocity/6(v-A) -> Fy-AFK/1, AccelDiff-v/1
  r x 3x2/1 -> abs-Ca/1
  Ca/1 -> r x 3x2/1
  r x 3x1/1 -> Cdx/1, Cdz/1, Cdy/1
  Cd/1 -> abs-Cd/1
  Cax/1 -> Fx-A/4
  Caz/1 -> Fz-A/4
  Fout/1 -> Force/1
  ForceCom/1 -> "r_{cg} x F"/2
  abs-Area/1 -> Ax/1, Az/1, Ay/1
  A x 3x3/1 -> abs-Area/1
  Cdz/1 -> Fz-w/4
  Cdx/1 -> Fx-V/4
  Ax/1 -> Fx-V/5
  Area/1 -> A x 3x3/1
  Az/1 -> Fz-w/5
  Fz-Sum/1 -> SwitchFz/3
  Fx-Sum/1 -> SwitchFx/3
  SwitchFx/1 -> ForceCom/1, Fout/1
  SwitchFz/1 -> Fout/3, ForceCom/3
  Zshift/1 -> SwitchFz/2, SwitchFx/2, SwitchFy/2
  VelDiff-u/1 -> V^2-u/2, V-u/1
  V-u/1 -> V^2-u/1
  3x3/1 -> r x 3x1/2, r x 3x2/2, r x 3x3/2, A x 3x3/2
  Mz/1 -> Fout/6
  My/1 -> Fout/5
  Mx/1 -> Fout/4
  "r_{cg} x F"/1 -> Mx/1, My/1, Mz/1
  Fz-AFK/1 -> Fz-Sum/3
  Fz-A/1 -> Fz-Sum/2
  Fz-w/1 -> Fz-Sum/1
  Fx-AFK/1 -> Fx-Sum/3
  Fx-A/1 -> Fx-Sum/2
  Fx-V/1 -> Fx-Sum/1
  OrbitalVelocity/4(w-A) -> AccelDiff-w/1, Fz-AFK/1
  AccelDiff-w/1 -> Fz-A/1
  Vol/1 -> Fx-A/3, Fz-A/2, Fx-AFK/2, Fz-AFK/2, Fy-AFK/2, Fy-A/2
  AccelDiff-u/1 -> Fx-A/1
  V^2-w/1 -> Fz-w/1
  Density/1 -> Fx-V/3, Fx-V1/3, Fz-w/3, Fx-A/2, Fz-A/3, Fx-AFK/3, Fz-AFK/3, Fy-AFK/3, Fy-A/3
  half/1 -> Fx-V/2, Fx-V1/2, Fz-w/2
  V^2-u/1 -> Fx-V/1
  VelDiff-w/1 -> V^2-w/2, V-w/1
  OrbitalVelocity/2(w-V) -> VelDiff-w/1
  OrbitalVelocity/1(u-V) -> VelDiff-u/1
  Uz/1 -> VelDiff-w/2
  Ux/1 -> VelDiff-u/2
  Uy/1 -> VelDiff-v/2
  Add Vel/1 -> Ux/1, Uz/1, Uy/1
  "dot{U}z"/1 -> AccelDiff-w/2
  OrbitalVelocity/3(u-A) -> Fx-AFK/1, AccelDiff-u/1
  "dot{U}x"/1 -> AccelDiff-u/2
  "dot{U}y"/1 -> AccelDiff-v/2
  ShiftCg/1 -> OrbitalVelocity/1(Disp), Zshift/1
  Disp-sl/1 -> ShiftCg/2
  r x 3x3/1 -> ShiftCg/1, "r_{cg} x F"/1
  Rotation3/1(rot[3,1-3]) -> 3x3/3
  Rotation1/1(rot[1,1-3]) -> 3x3/1
  Rotation2/1(rot[2,1-3]) -> 3x3/2
  rot2/1 -> Rotation1/2(rot2), Rotation2/2(rot2), Rotation3/2(rot2)
  rot1/1 -> Rotation1/1(rot1), Rotation2/1(rot1), Rotation3/1(rot1)
  rot3/1 -> Rotation1/3(rot3), Rotation2/3(rot3)
  Disp-sr/1 -> rot1/1, rot2/1, rot3/1
  Disp/1 -> Disp-sr/1, Disp-sl/1
  Vel-sl/1 -> Add Vel/1
  Add Accel/1 -> "dot{U}x"/1, "dot{U}y"/1, "dot{U}z"/1
  Accel-sl/1 -> Add Accel/3
  "dot{w} x r2"/1 -> Add Accel/2
  Accel-sr/1 -> "dot{w} x r2"/1
  Accel/1 -> Accel-sr/1, Accel-sl/1
  r/1 -> w x r/2, "dot{w} x r2"/2, r x 3x3/1
  "Vel-sr "/1 -> w x r/1, w x w x r/1
  w x w x r/1 -> Add Accel/1
  w x r/1 -> w x w x r/2, Add Vel/2
  Vel/1 -> "Vel-sr "/1, Vel-sl/1

== system RM3ControlSim/Rigid Body/Hydrodynamic Body/Morrison Element and ViscousDampingForceCalculation/Morrison Element Variant Subsystem/Morrison Element On/Irregular Wave Morison Force/MorrisonElements/MorisonElementIrregular ==
  Disp : Inport
  waves.kirr : Inport  Port=2  Partition=on  PartitionDimension=1  PartitionWidth=1
  waves.w : Inport  Port=3  Partition=on  PartitionDimension=1  PartitionWidth=1
  waves.A : Inport  Port=4  Partition=on  PartitionDimension=1  PartitionWidth=1
  waves.RandPhase : Inport  Port=5  Partition=on  PartitionDimension=1  PartitionWidth=1
  Time : Inport  Port=6
  For Each : ForEach  DisableCoverage=on  IndexMode=One-based
  MATLAB Function : MATLAB Function  TreatAsAtomicUnit=on
  gravity : Constant  Value=simu.g  VectorParams1D=off
  rampTime : Constant  Value=simu.rampTime  VectorParams1D=off
  waterDepth : Constant  Value=waves.waterDepth  VectorParams1D=off
  waveDirection : Constant  Value=waves.waveDir  VectorParams1D=off
  u-V : Outport  ConcatenationDimension=1
  w-V : Outport  Port=2  ConcatenationDimension=1
  x-A : Outport  Port=3  ConcatenationDimension=1
  w-A : Outport  Port=4  ConcatenationDimension=1
  v-V : Outport  Port=5  ConcatenationDimension=1
  y-A : Outport  Port=6  ConcatenationDimension=1
  wires:
  MATLAB Function/3(w) -> w-V/1
  MATLAB Function/4(xa) -> x-A/1
  MATLAB Function/6(za) -> w-A/1
  MATLAB Function/5(ya) -> y-A/1
  MATLAB Function/2(v) -> v-V/1
  Time/1 -> MATLAB Function/6(time)
  waves.kirr/1 -> MATLAB Function/2(waveNumber)
  MATLAB Function/1(u) -> u-V/1
  waves.RandPhase/1 -> MATLAB Function/5(randPhase)
  waves.A/1 -> MATLAB Function/4(waveAmp)
  waves.w/1 -> MATLAB Function/3(waveFreq)
  Disp/1 -> MATLAB Function/1(disp)
  rampTime/1 -> MATLAB Function/7(rampT)
  waveDirection/1 -> MATLAB Function/8(waveDir)
  waterDepth/1 -> MATLAB Function/9(waterDepth)
  gravity/1 -> MATLAB Function/10(g)

== system RM3ControlSim/Rigid Body/Hydrodynamic Body/Morrison Element and ViscousDampingForceCalculation/Morrison Element Variant Subsystem/Morrison Element On/Irregular Wave Morison Force/MorrisonElements/Rotation1 ==
  rot1 : Inport
  rot2 : Inport  Port=2
  rot3 : Inport  Port=3
  2 : Product
  3 : Product  Inputs=3
  7 : Product
  8 : Product  Inputs=3
  Combine : Concatenate  NumInputs=3  Mode=Multidimensional array  ConcatenateDimension=2
  Trigonometric Function{,1..2,6,9,11} (6 alike) : Trigonometry  Operator=cos
  Trigonometric Function{3..5,7..8,10} (6 alike) : Trigonometry
  rot11 : Product
  rot12 : Sum
  rot13 : Sum  Inputs=+-
  rot[1,1-3] : Outport
  wires:
  rot13/1 -> Combine/3
  8/1 -> rot13/2
  7/1 -> rot13/1
  Trigonometric Function11/1 -> 8/3
  Trigonometric Function10/1 -> 8/2
  Trigonometric Function9/1 -> 8/1
  Trigonometric Function8/1 -> 7/2
  Trigonometric Function7/1 -> 7/1
  rot1/1 -> Trigonometric Function7/1, Trigonometric Function9/1, Trigonometric Function4/1, Trigonometric Function2/1
  rot3/1 -> Trigonometric Function8/1, Trigonometric Function11/1, Trigonometric Function6/1, Trigonometric Function3/1, Trigonometric Function1/1
  rot2/1 -> Trigonometric Function10/1, Trigonometric Function5/1, Trigonometric Function/1
  Combine/1 -> rot[1,1-3]/1
  rot12/1 -> Combine/2
  3/1 -> rot12/2
  2/1 -> rot12/1
  Trigonometric Function6/1 -> 3/3
  Trigonometric Function5/1 -> 3/2
  Trigonometric Function4/1 -> 3/1
  Trigonometric Function3/1 -> 2/2
  Trigonometric Function2/1 -> 2/1
  rot11/1 -> Combine/1
  Trigonometric Function1/1 -> rot11/2
  Trigonometric Function/1 -> rot11/1

== system RM3ControlSim/Rigid Body/Hydrodynamic Body/Morrison Element and ViscousDampingForceCalculation/Morrison Element Variant Subsystem/Morrison Element On/Irregular Wave Morison Force/MorrisonElements/Rotation2 ==
  rot1 : Inport
  rot2 : Inport  Port=2
  rot3 : Inport  Port=3
  2 : Product
  3 : Product  Inputs=3
  7 : Product
  8 : Product  Inputs=3
  Combine : Concatenate  NumInputs=3  Mode=Multidimensional array  ConcatenateDimension=2
  Gain : Gain  Gain=-1
  Trigonometric Function{,2..3,8..9} (5 alike) : Trigonometry  Operator=cos
  Trigonometric Function{1,4..7,10..11} (7 alike) : Trigonometry
  rot11 : Product
  rot12 : Sum  Inputs=+-
  rot13 : Sum
  rot[2,1-3] : Outport
  wires:
  Gain/1 -> rot11/1
  rot13/1 -> Combine/3
  8/1 -> rot13/2
  7/1 -> rot13/1
  Trigonometric Function11/1 -> 8/3
  Trigonometric Function10/1 -> 8/2
  Trigonometric Function9/1 -> 8/1
  Trigonometric Function8/1 -> 7/2
  Trigonometric Function7/1 -> 7/1
  rot1/1 -> Trigonometric Function7/1, Trigonometric Function9/1, Trigonometric Function4/1, Trigonometric Function2/1
  rot3/1 -> Trigonometric Function8/1, Trigonometric Function11/1, Trigonometric Function6/1, Trigonometric Function3/1, Trigonometric Function1/1
  rot2/1 -> Trigonometric Function10/1, Trigonometric Function5/1, Trigonometric Function/1
  Combine/1 -> rot[2,1-3]/1
  rot12/1 -> Combine/2
  3/1 -> rot12/2
  2/1 -> rot12/1
  Trigonometric Function6/1 -> 3/3
  Trigonometric Function5/1 -> 3/2
  Trigonometric Function4/1 -> 3/1
  Trigonometric Function3/1 -> 2/2
  Trigonometric Function2/1 -> 2/1
  rot11/1 -> Combine/1
  Trigonometric Function1/1 -> rot11/2
  Trigonometric Function/1 -> Gain/1

== system RM3ControlSim/Rigid Body/Hydrodynamic Body/Morrison Element and ViscousDampingForceCalculation/Morrison Element Variant Subsystem/Morrison Element On/Irregular Wave Morison Force/MorrisonElements/Rotation3 ==
  rot1 : Inport
  rot2 : Inport  Port=2
  2 : Product
  7 : Product
  Combine : Concatenate  NumInputs=3  Mode=Multidimensional array  ConcatenateDimension=2
  Gain1 : Gain  Gain=-1
  TrigFun1 : Trigonometry
  TrigFun2 : Trigonometry
  TrigFun3 : Trigonometry  Operator=cos
  TrigFun4 : Trigonometry  Operator=cos
  TrigFun5 : Trigonometry  Operator=cos
  rot[3,1-3] : Outport
  wires:
  Gain1/1 -> 2/1
  TrigFun2/1 -> Gain1/1
  7/1 -> Combine/3
  rot1/1 -> TrigFun4/1, TrigFun2/1
  TrigFun5/1 -> 7/2
  TrigFun4/1 -> 7/1
  rot2/1 -> TrigFun1/1, TrigFun3/1, TrigFun5/1
  Combine/1 -> rot[3,1-3]/1
  2/1 -> Combine/2
  TrigFun3/1 -> 2/2
  TrigFun1/1 -> Combine/1

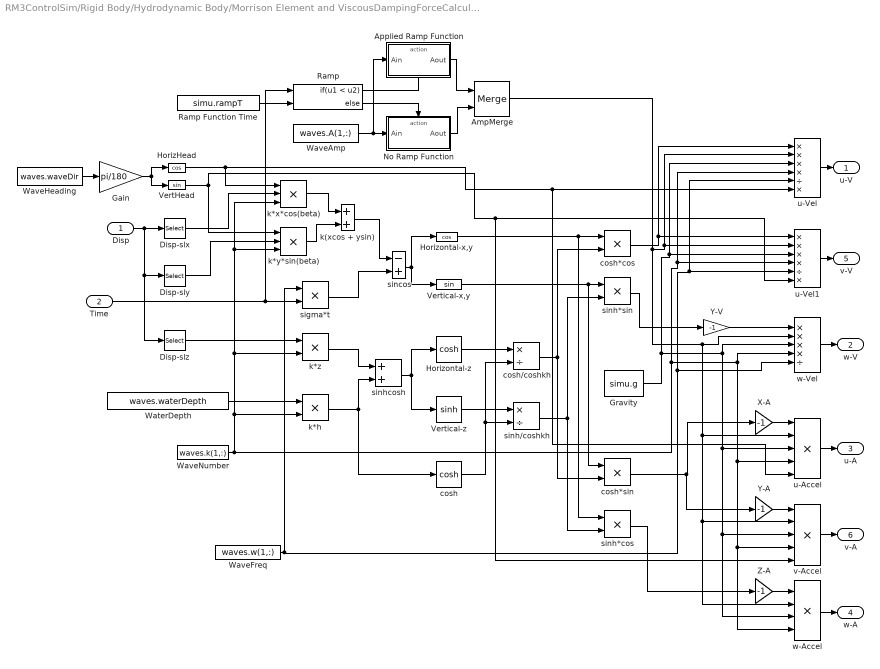
== system RM3ControlSim/Rigid Body/Hydrodynamic Body/Morrison Element and ViscousDampingForceCalculation/Morrison Element Variant Subsystem/Morrison Element On/No Wave Morison Force/MorrisonElements/OrbitalVelocity ==
  Disp : Inport
  Time : Inport  Port=2
  AmpMerge : Merge
  Applied Ramp Function : Subsystem  TreatAsAtomicUnit=on
  Disp-slx : Selector  InputPortWidth=3  IndexOptions=Index vector (dialog)  Indices=[1]  OutputSizes=1
  Disp-sly : Selector  InputPortWidth=3  IndexOptions=Index vector (dialog)  Indices=[2]  OutputSizes=1
  Disp-slz : Selector  InputPortWidth=3  IndexOptions=Index vector (dialog)  Indices=[3]  OutputSizes=1
  Gain : Gain  Gain=pi/180
  Gravity : Constant  Value=simu.g
  HorizHead : Trigonometry  Operator=cos
  Horizontal-x,y : Trigonometry  Operator=cos
  Horizontal-z : Trigonometry  Operator=cosh
  No Ramp Function : Subsystem  TreatAsAtomicUnit=on
  Ramp : If  NumInputs=2  IfExpression=u1 < u2
  Ramp Function Time : Constant  Value=simu.rampT
  VertHead : Trigonometry
  Vertical-x,y : Trigonometry
  Vertical-z : Trigonometry  Operator=sinh
  WaterDepth : Constant  Value=waves.waterDepth
  WaveAmp : Constant  Value=waves.A(1,:)
  WaveFreq : Constant  Value=waves.w(1,:)
  WaveHeading : Constant  Value=waves.waveDir
  WaveNumber : Constant  Value=waves.k(1,:)
  X-A : Gain  Gain=-1
  Y-A : Gain  Gain=-1
  Y-V : Gain  Gain=-1
  Z-A : Gain  Gain=-1
  cosh : Trigonometry  Operator=cosh
  cosh*cos : Product  Inputs=**
  cosh*sin : Product  Inputs=**
  cosh/coshkh : Product  Inputs=*/
  k(xcos + ysin) : Sum
  k*h : Product
  k*x*cos(beta) : Product  Inputs=3
  k*y*sin(beta) : Product  Inputs=3
  k*z : Product
  sigma*t : Product
  sincos : Sum  Inputs=-+
  sinh*cos : Product  Inputs=**
  sinh*sin : Product  Inputs=**
  sinh/coshkh : Product  Inputs=*/
  sinhcosh : Sum
  u-Accel : Product  Inputs=*****
  u-Vel : Product  Inputs=****/*
  u-Vel1 : Product  Inputs=****/*
  v-Accel : Product  Inputs=*****
  w-Accel : Product  Inputs=****
  w-Vel : Product  Inputs=****/
  u-V : Outport
  w-V : Outport  Port=2
  u-A : Outport  Port=3
  w-A : Outport  Port=4
  v-V : Outport  Port=5
  v-A : Outport  Port=6
  wires:
  v-Accel/1 -> v-A/1
  Y-A/1 -> v-Accel/1
  u-Vel/1 -> u-V/1
  u-Vel1/1 -> v-V/1
  k(xcos + ysin)/1 -> sincos/1
  k*x*cos(beta)/1 -> k(xcos + ysin)/1
  k*y*sin(beta)/1 -> k(xcos + ysin)/2
  VertHead/1 -> v-Accel/5, u-Vel1/6, k*y*sin(beta)/1
  HorizHead/1 -> k*x*cos(beta)/1, u-Vel/6, u-Accel/5
  Disp-slx/1 -> k*x*cos(beta)/2
  Gain/1 -> VertHead/1, HorizHead/1
  WaveHeading/1 -> Gain/1
  WaveAmp/1 -> No Ramp Function/1(Ain), Applied Ramp Function/1(Ain)
  WaveFreq/1 -> sigma*t/1, u-Vel/5, u-Vel1/5, w-Vel/5
  Disp-slz/1 -> k*z/1
  Applied Ramp Function/1(Aout) -> AmpMerge/1
  No Ramp Function/1(Aout) -> AmpMerge/2
  Time/1 -> sigma*t/2, Ramp/1
  Ramp/1 -> Applied Ramp Function/Action
  Ramp/2 -> No Ramp Function/Action
  Ramp Function Time/1 -> Ramp/2
  sinh*cos/1 -> Z-A/1
  cosh*sin/1 -> X-A/1, Y-A/1
  w-Accel/1 -> w-A/1
  u-Accel/1 -> u-A/1
  w-Vel/1 -> w-V/1
  Z-A/1 -> w-Accel/1
  X-A/1 -> u-Accel/1
  Y-V/1 -> w-Vel/1
  sinh*sin/1 -> Y-V/1
  Gravity/1 -> u-Vel/3, u-Vel1/3, u-Accel/3, w-Accel/3, v-Accel/3, w-Vel/3
  AmpMerge/1 -> u-Vel/2, u-Vel1/2, u-Accel/2, v-Accel/2, w-Accel/2, w-Vel/2
  cosh*cos/1 -> u-Vel/1, u-Vel1/1
  Disp-sly/1 -> k*y*sin(beta)/2
  cosh/coshkh/1 -> cosh*sin/2, cosh*cos/2
  Horizontal-x,y/1 -> cosh*cos/1, sinh*cos/1
  sinh/coshkh/1 -> sinh*sin/2, sinh*cos/2
  Vertical-x,y/1 -> sinh*sin/1, cosh*sin/1
  Vertical-z/1 -> sinh/coshkh/1
  cosh/1 -> cosh/coshkh/2, sinh/coshkh/2
  Horizontal-z/1 -> cosh/coshkh/1
  sinhcosh/1 -> Horizontal-z/1, Vertical-z/1
  k*h/1 -> sinhcosh/2, cosh/1
  k*z/1 -> sinhcosh/1
  sincos/1 -> Horizontal-x,y/1, Vertical-x,y/1
  sigma*t/1 -> sincos/2
  WaterDepth/1 -> k*h/1
  WaveNumber/1 -> u-Vel/4, u-Vel1/4, u-Accel/4, w-Accel/4, v-Accel/4, w-Vel/4, k*x*cos(beta)/3, k*y*sin(beta)/3, k*z/2, k*h/2
  Disp/1 -> Disp-slx/1, Disp-sly/1, Disp-slz/1

== system RM3ControlSim/Rigid Body/Hydrodynamic Body/Morrison Element and ViscousDampingForceCalculation/Morrison Element Variant Subsystem/Morrison Element On/No Wave Morison Force/MorrisonElements/Rotation1 ==
  rot1 : Inport
  rot2 : Inport  Port=2
  rot3 : Inport  Port=3
  2 : Product
  3 : Product  Inputs=3
  7 : Product
  8 : Product  Inputs=3
  Combine : Concatenate  NumInputs=3  Mode=Multidimensional array  ConcatenateDimension=2
  Trigonometric Function{,1..2,6,9,11} (6 alike) : Trigonometry  Operator=cos
  Trigonometric Function{3..5,7..8,10} (6 alike) : Trigonometry
  rot11 : Product
  rot12 : Sum
  rot13 : Sum  Inputs=+-
  rot[1,1-3] : Outport
  wires:
  rot13/1 -> Combine/3
  8/1 -> rot13/2
  7/1 -> rot13/1
  Trigonometric Function11/1 -> 8/3
  Trigonometric Function10/1 -> 8/2
  Trigonometric Function9/1 -> 8/1
  Trigonometric Function8/1 -> 7/2
  Trigonometric Function7/1 -> 7/1
  rot1/1 -> Trigonometric Function7/1, Trigonometric Function9/1, Trigonometric Function4/1, Trigonometric Function2/1
  rot3/1 -> Trigonometric Function8/1, Trigonometric Function11/1, Trigonometric Function6/1, Trigonometric Function3/1, Trigonometric Function1/1
  rot2/1 -> Trigonometric Function10/1, Trigonometric Function5/1, Trigonometric Function/1
  Combine/1 -> rot[1,1-3]/1
  rot12/1 -> Combine/2
  3/1 -> rot12/2
  2/1 -> rot12/1
  Trigonometric Function6/1 -> 3/3
  Trigonometric Function5/1 -> 3/2
  Trigonometric Function4/1 -> 3/1
  Trigonometric Function3/1 -> 2/2
  Trigonometric Function2/1 -> 2/1
  rot11/1 -> Combine/1
  Trigonometric Function1/1 -> rot11/2
  Trigonometric Function/1 -> rot11/1

== system RM3ControlSim/Rigid Body/Hydrodynamic Body/Morrison Element and ViscousDampingForceCalculation/Morrison Element Variant Subsystem/Morrison Element On/No Wave Morison Force/MorrisonElements/Rotation2 ==
  rot1 : Inport
  rot2 : Inport  Port=2
  rot3 : Inport  Port=3
  2 : Product
  3 : Product  Inputs=3
  7 : Product
  8 : Product  Inputs=3
  Combine : Concatenate  NumInputs=3  Mode=Multidimensional array  ConcatenateDimension=2
  Gain : Gain  Gain=-1
  Trigonometric Function{,2..3,8..9} (5 alike) : Trigonometry  Operator=cos
  Trigonometric Function{1,4..7,10..11} (7 alike) : Trigonometry
  rot11 : Product
  rot12 : Sum  Inputs=+-
  rot13 : Sum
  rot[2,1-3] : Outport
  wires:
  Gain/1 -> rot11/1
  rot13/1 -> Combine/3
  8/1 -> rot13/2
  7/1 -> rot13/1
  Trigonometric Function11/1 -> 8/3
  Trigonometric Function10/1 -> 8/2
  Trigonometric Function9/1 -> 8/1
  Trigonometric Function8/1 -> 7/2
  Trigonometric Function7/1 -> 7/1
  rot1/1 -> Trigonometric Function7/1, Trigonometric Function9/1, Trigonometric Function4/1, Trigonometric Function2/1
  rot3/1 -> Trigonometric Function8/1, Trigonometric Function11/1, Trigonometric Function6/1, Trigonometric Function3/1, Trigonometric Function1/1
  rot2/1 -> Trigonometric Function10/1, Trigonometric Function5/1, Trigonometric Function/1
  Combine/1 -> rot[2,1-3]/1
  rot12/1 -> Combine/2
  3/1 -> rot12/2
  2/1 -> rot12/1
  Trigonometric Function6/1 -> 3/3
  Trigonometric Function5/1 -> 3/2
  Trigonometric Function4/1 -> 3/1
  Trigonometric Function3/1 -> 2/2
  Trigonometric Function2/1 -> 2/1
  rot11/1 -> Combine/1
  Trigonometric Function1/1 -> rot11/2
  Trigonometric Function/1 -> Gain/1

== system RM3ControlSim/Rigid Body/Hydrodynamic Body/Morrison Element and ViscousDampingForceCalculation/Morrison Element Variant Subsystem/Morrison Element On/No Wave Morison Force/MorrisonElements/Rotation3 ==
  rot1 : Inport
  rot2 : Inport  Port=2
  2 : Product
  7 : Product
  Combine : Concatenate  NumInputs=3  Mode=Multidimensional array  ConcatenateDimension=2
  Gain1 : Gain  Gain=-1
  TrigFun1 : Trigonometry
  TrigFun2 : Trigonometry
  TrigFun3 : Trigonometry  Operator=cos
  TrigFun4 : Trigonometry  Operator=cos
  TrigFun5 : Trigonometry  Operator=cos
  rot[3,1-3] : Outport
  wires:
  Gain1/1 -> 2/1
  TrigFun2/1 -> Gain1/1
  7/1 -> Combine/3
  rot1/1 -> TrigFun4/1, TrigFun2/1
  TrigFun5/1 -> 7/2
  TrigFun4/1 -> 7/1
  rot2/1 -> TrigFun1/1, TrigFun3/1, TrigFun5/1
  Combine/1 -> rot[3,1-3]/1
  2/1 -> Combine/2
  TrigFun3/1 -> 2/2
  TrigFun1/1 -> Combine/1
